simulink model "Assignment1"  (R2020a)
settings: Solver=FixedStepAuto  StartTime=0.0  StopTime=10.0  FixedStep=1e-3  RelTol=1e-3  EnableMultiTasking=on
undefined symbols (not defined in the file or in its folder): D0, D1, D10, D11, D12, D13, D2, D3, D4, D5, D6, D7, D8, D9, PTA0, PTA1, PTA2, PTB23, PTB9, PTC16, PTC17, PTC2, PTC3, PTC4, PTD0, PTD1, PTD2, PTD3
libraries: frdmk64flib x24
settings Model: ExtModeTrigDuration=5  Creator=iceca  LastModifiedBy=iceca
settings OptimizationCC: EnhancedBackFolding=on  PassReuseOutputArgsAs=Individual arguments  ZeroExternalMemoryAtStartup=off  ZeroInternalMemoryAtStartup=off  MaxStackSize=64  OptimizeBlockOrder=speed  DifferentSizesBufferReuse=on  OptimizationCustomize=off  EfficientTunableParamExpr=on
settings DebuggingCC: ParameterTunabilityLossMsg=error
settings HardwareCC: ProdBitPerPointer=32  ProdBitPerSizeT=32  ProdBitPerPtrDiffT=32  ProdLargestAtomicInteger=Long  ProdLargestAtomicFloat=Double  ProdWordSize=32  ProdHWDeviceType=ARM Compatible->ARM Cortex
settings SFSimCC: MATLABDynamicMemAlloc=off
settings RTWCC: SystemTargetFile=ert.tlc  HardwareBoard=NXP FRDM-K64F  TemplateMakefile=ert_default_tmf  Toolchain=GNU Tools for ARM Embedded Processors
settings CodeAppCC: ForceParamTrailComments=on  IgnoreCustomStorageClasses=off  OperatorAnnotations=on  SimulinkDataObjDesc=on  SFDataObjDesc=on  InsertBlockDesc=on

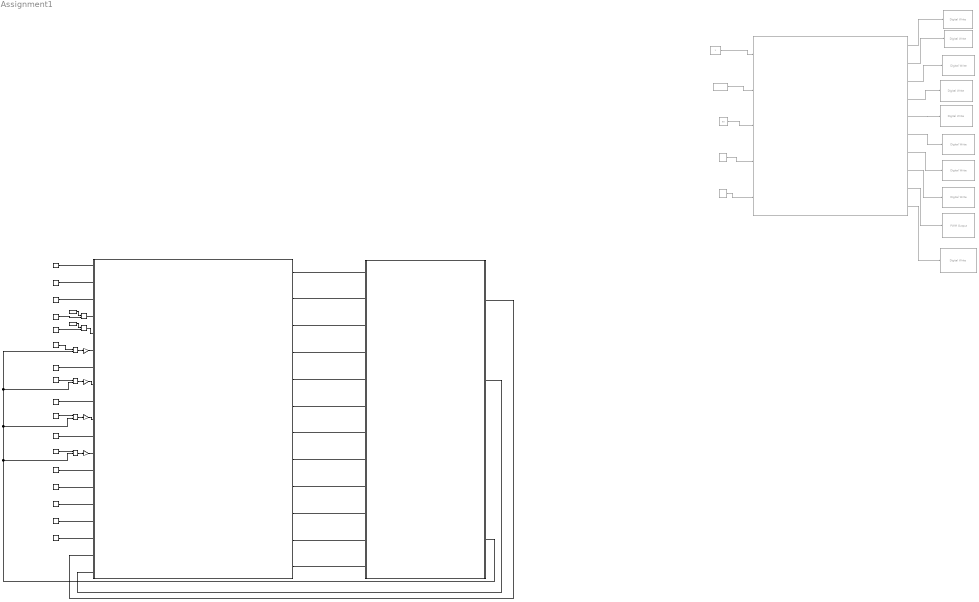
== system Assignment1 ==
  note: Domain: OFF, or percentage
      | in the set (3, 6, 9, 12, 15, 18, 21,25)
  note: Units: pace per minute(ppm)
  note: Domain: 1=Atrial, 2=Ventricular
  note: HARDWARE
  note: Domain: 0=None, 1=Atrial, 2=Ventricular
  note: Domain: 0=None, 2=Inhibited
  note: Units: V
  note: Units: msec
  note: Units: V
  note: Units: msec
  note: Units: V
  note: Units: msec
  note: Units: msec
  note: Units: V
  note: Units: msec
  note: Domain:true, false
  note: Units: msec
  note: Units: pace per minute(ppm)
  note: STATEFLOW
  ARP : Constant  Value=250
  Atrial_Amplitude : Constant  Value=1.5
  Atrial_Pulse_Width : Constant  Value=20
  Atrial_Sensitivity : Constant  Value=3.5
  Chart : Stateflow chart  Commented=on  TreatAsAtomicUnit=on
  Chart1 : Stateflow chart  TreatAsAtomicUnit=on
  Constant24 : Constant  Commented=on  Value=60
  Constant25 : Constant  Commented=on  Value=3.7
  Constant26 : Constant  Commented=on  Value=120
  Constant27 : Constant  Commented=on  Value=10
  Constant28 : Constant  Commented=on
  Digital Write24 : frdmk64flib/Digital Write  Commented=on  Whichpin=PTB9 (D2)
  Digital Write25 : frdmk64flib/Digital Write  Commented=on  Whichpin=PTD0 (D10)
  Digital Write26 : frdmk64flib/Digital Write  Commented=on  Whichpin=PTA0 (D8)
  Digital Write27 : frdmk64flib/Digital Write  Commented=on  Whichpin=PTD2 (D11)
  Digital Write28 : frdmk64flib/Digital Write  Commented=on  Whichpin=PTB23 (D4)
  Digital Write29 : frdmk64flib/Digital Write  Commented=on  Whichpin=PTC3 (D7)
  Digital Write30 : frdmk64flib/Digital Write  Commented=on  Whichpin=PTC4 (D9)
  Digital Write31 : frdmk64flib/Digital Write  Commented=on  Whichpin=PTD3 (D12)
  Digital Write32 : frdmk64flib/Digital Write  Commented=on  Whichpin=BLUE_LED
  Divide{,1..5} (6 alike) : Product  Inputs=*/
  Gain{,1..3} (4 alike) : Gain  Gain=100
  Hysterisis : Constant  Value=0
  Hysterisis Escape Interval : Constant  Value=10
  Lower_Rate_Limit : Constant  Value=60
  Mode_Chamber_Paced : Constant  Value=2
  Mode_Chamber_Sensed : Constant  Value=2
  Mode_Response : Constant  Value=2
  PVARP : Constant  Value=250
  PWM Output : frdmk64flib/PWM Output  Commented=on  Whichpin=PTA2 (D5)  InitialFrequency=2000  InitialDutyCycle=50
  Rate_Smoothing : Constant
  Subsystem : Subsystem
  Upper_Rate_Limit : Constant  Value=120
  VRP : Constant  Value=250
  Ventricular_Amplitude : Constant  Value=4
  Ventricular_Pulse_Width : Constant  Value=10
  Ventricular_Sensitivity : Constant  Value=4
  msec/minute : Constant  Value=60000
  msec/minute 1 : Constant  Value=60000
  wires:
  Chart/1(PACE_CHARGE_CTRL_D2) -> Digital Write24/1
  Chart/2(PACE_GND_CTRL_D10) -> Digital Write25/1
  Chart/3(ATR_PACE_CTRL_D8) -> Digital Write26/1
  Chart/4(ATR_GND_CTRL_D11) -> Digital Write27/1
  Chart/5(Z_ATR_CTRL_D4) -> Digital Write28/1
  Chart/6(Z_VENT_CTRL_D7) -> Digital Write29/1
  Chart/7(VENT_GND_CTRL_D12) -> Digital Write31/1
  Chart/8(VENT_PACE_CTRL_D9) -> Digital Write30/1
  Chart/9(PACING_REF_PWM_D5) -> PWM Output/1
  Constant28/1 -> Chart/1(Pacing_Mode)
  Constant25/1 -> Chart/5(Pulse_Amplitude)
  Constant26/1 -> Chart/4(Upper_Rate_Limit)
  Constant24/1 -> Chart/3(Lower_Rate_Limit)
  Constant27/1 -> Chart/2(Pulse_Width)
  Chart/10(LED_RED) -> Digital Write32/1
  Gain1/1 -> Chart1/10(Atrial_Amplitude)
  VRP/1 -> Chart1/9(VRP)
  Atrial_Sensitivity/1 -> Divide3/1
  Divide2/1 -> Gain1/1
  Divide1/1 -> Gain2/1
  Atrial_Amplitude/1 -> Divide2/1
  Ventricular_Amplitude/1 -> Divide/1
  Ventricular_Sensitivity/1 -> Divide1/1
  Mode_Chamber_Paced/1 -> Chart1/1(Mode_Chamber_Paced)
  Divide3/1 -> Gain3/1
  Gain3/1 -> Chart1/12(Atrial_Sensitivity)
  Gain2/1 -> Chart1/8(Ventricular_Sensitivity)
  Mode_Response/1 -> Chart1/3(Mode_Response)
  Subsystem/4(VOLTAGE_LOGIC_LEVEL) -> Divide3/2, Divide2/2, Divide1/2, Divide/2
  Ventricular_Pulse_Width/1 -> Chart1/7(Ventricular_Pulse_Width)
  Rate_Smoothing/1 -> Chart1/15(Rate_Smoothing)
  Divide/1 -> Gain/1
  Mode_Chamber_Sensed/1 -> Chart1/2(Mode_Chamber_Sensed)
  Atrial_Pulse_Width/1 -> Chart1/11(Atrial_Pulse_Width)
  Hysterisis/1 -> Chart1/16(Hysterisis)
  ARP/1 -> Chart1/13(ARP)
  Gain/1 -> Chart1/6(Ventricular_Amplitude)
  PVARP/1 -> Chart1/14(PVARP)
  msec/minute/1 -> Divide4/1
  Lower_Rate_Limit/1 -> Divide4/2
  Divide4/1 -> Chart1/4(Lower_Rate_Limit)
  Upper_Rate_Limit/1 -> Divide5/2
  msec/minute 1/1 -> Divide5/1
  Divide5/1 -> Chart1/5(Upper_Rate_Limit)
  Hysterisis Escape Interval/1 -> Chart1/17(Hysterisis_Escape_Interval)
  Chart1/1(PACE_CHARGE_CTRL) -> Subsystem/1(PACE_CHARGE_CTRL)
  Chart1/2(PACE_GND_CTRL) -> Subsystem/2(PACE_GND_CTRL)
  Chart1/3(PACING_REF_PWM) -> Subsystem/3(PACING_REF_PWM)
  Chart1/4(VENT_PACE_CTRL) -> Subsystem/4(VENT_PACE_CTRL)
  Chart1/5(ATR_PACE_CTRL) -> Subsystem/5(ATR_PACE_CTRL)
  Chart1/6(ATR_GND_CTRL) -> Subsystem/6(ATR_GND_CTRL)
  Chart1/7(Z_ATR_CTRL) -> Subsystem/7(Z_ATR_CTRL)
  Chart1/8(Z_VENT_CTRL) -> Subsystem/8(Z_VENT_CTRL)
  Chart1/9(VENT_GND_CTRL) -> Subsystem/9(VENT_GND_CTRL)
  Chart1/10(FRONT_END_CTRL) -> Subsystem/10(FRONT_END_CTRL)
  Chart1/11(ATR_CMP_REF_PWM) -> Subsystem/11(ATR_CMP_REF_PWM)
  Chart1/12(VENT_CMP_REF_PWM) -> Subsystem/12(VENT_CMP_REF_PWM)
  Subsystem/1(VENT_CMP_DETECT) -> Chart1/18(ATR_CMP_DETECT)
  Subsystem/2(ATR_CMP_DETECT) -> Chart1/19(VENT_CMP_DETECT)

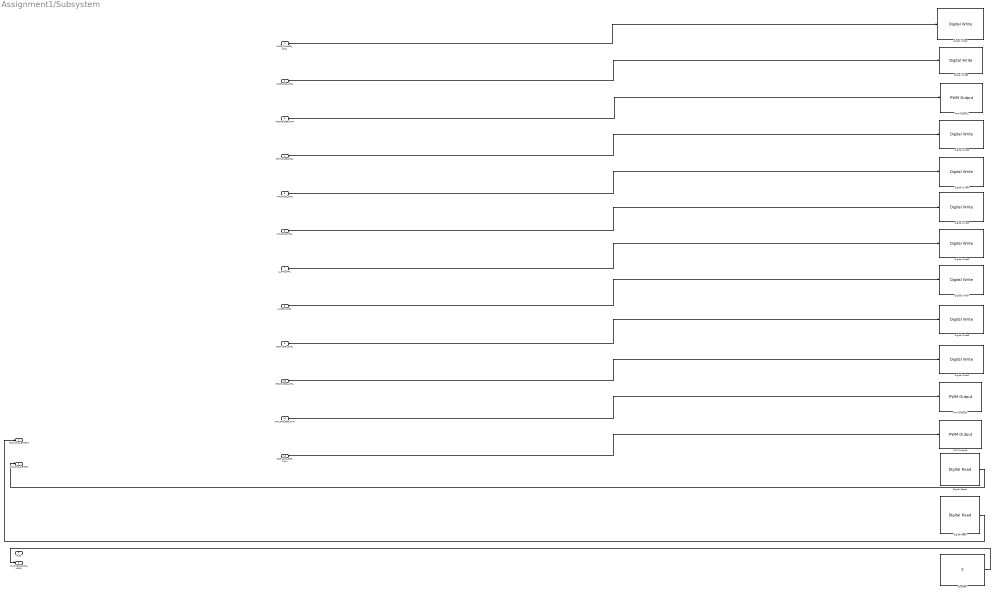
== system Assignment1/Subsystem ==
  PACE_CHARGE_CTRL : Inport
  PACE_GND_CTRL : Inport  Port=2
  PACING_REF_PWM : Inport  Port=3
  VENT_PACE_CTRL : Inport  Port=4
  ATR_PACE_CTRL : Inport  Port=5
  ATR_GND_CTRL : Inport  Port=6
  Z_ATR_CTRL : Inport  Port=7
  Z_VENT_CTRL : Inport  Port=8
  VENT_GND_CTRL : Inport  Port=9
  FRONT_END_CTRL : Inport  Port=10
  ATR_CMP_REF_PWM : Inport  Port=11
  VENT_CMP_REF_PWM : Inport  Port=12
  Constant : Constant  Value=5
  Digital Read : frdmk64flib/Digital Read  Whichpin=PTC16 (D0)  SampleTime=-1
  Digital Read1 : frdmk64flib/Digital Read  Whichpin=PTC17 (D1)  SampleTime=-1
  Digital Write1 : frdmk64flib/Digital Write  Whichpin=PTD1 (D13)
  Digital Write2 : frdmk64flib/Digital Write  Whichpin=PTB9 (D2)
  Digital Write3 : frdmk64flib/Digital Write  Whichpin=PTD0 (D10)
  Digital Write4 : frdmk64flib/Digital Write  Whichpin=PTA0 (D8)
  Digital Write5 : frdmk64flib/Digital Write  Whichpin=PTD2 (D11)
  Digital Write6 : frdmk64flib/Digital Write  Whichpin=PTB23 (D4)
  Digital Write7 : frdmk64flib/Digital Write  Whichpin=PTC3 (D7)
  Digital Write8 : frdmk64flib/Digital Write  Whichpin=PTC4 (D9)
  Digital Write9 : frdmk64flib/Digital Write  Whichpin=PTD3 (D12)
  PWM Output1 : frdmk64flib/PWM Output  Whichpin=PTA2 (D5)  InitialFrequency=2000  InitialDutyCycle=0
  PWM Output2 : frdmk64flib/PWM Output  Whichpin=PTC2 (D6)  InitialFrequency=2000  InitialDutyCycle=0
  PWM Output3 : frdmk64flib/PWM Output  Whichpin=PTA1 (D3)  InitialFrequency=2000  InitialDutyCycle=0
  VENT_CMP_DETECT : Outport
  ATR_CMP_DETECT : Outport  Port=2
  Out3 : Outport  Port=3
  VOLTAGE_LOGIC_LEVEL : Outport  Port=4
  wires:
  PACING_REF_PWM/1 -> PWM Output1/1
  VENT_GND_CTRL/1 -> Digital Write9/1
  PACE_GND_CTRL/1 -> Digital Write3/1
  ATR_GND_CTRL/1 -> Digital Write5/1
  ATR_CMP_REF_PWM/1 -> PWM Output2/1
  VENT_PACE_CTRL/1 -> Digital Write8/1
  Digital Read1/1 -> ATR_CMP_DETECT/1
  Digital Read/1 -> VENT_CMP_DETECT/1
  VENT_CMP_REF_PWM/1 -> PWM Output3/1
  Z_VENT_CTRL/1 -> Digital Write7/1
  Z_ATR_CTRL/1 -> Digital Write6/1
  PACE_CHARGE_CTRL/1 -> Digital Write2/1
  ATR_PACE_CTRL/1 -> Digital Write4/1
  FRONT_END_CTRL/1 -> Digital Write1/1
  Constant/1 -> VOLTAGE_LOGIC_LEVEL/1

== stateflow chart Assignment1/Chart1 ==
  note: |
  note: |
  note: 3 Sections: Atrial only States | Common States | Ventricular only States
  note: |
  note: |
  state Charging_C22
    entry:
    ATR_PACE_CTRL   = LOW;
    VENT_PACE_CTRL = LOW;
  note: Phase 1:
      | Charging Capacitors
  state Atrial_Charge
    entry:
    PACING_REF_PWM = Atrial_Amplitude;
  state Ventricular_Charge
    entry:
    PACING_REF_PWM = Ventricular_Amplitude;
  note: ----------------------------------------------------------------------------------
  state Discharging_C21_and_Pace_Interval_Calculations
    entry:
    PACE_CHARGE_CTRL = HIGH;
    %Discharging C21
    PACE_GND_CTRL=HIGH;
    VENT_PACE_CTRL=LOW;
    Z_ATR_CTRL= LOW;
    Z_VENT_CTRL = LOW;
    ATR_PACE_CTRL = LOW;
    Pace_Interval = Lower_Rate_Limit;
    if Hysterisis == HIGH
    Pace_Interval = Pace_Interval + Hysterisis_Escape_Interval;
    end
  note: Phase 2:
      | Discharging Capacitors
  state Atrial_Discharge
    entry:
    ATR_GND_CTRL= HIGH;
    VENT_GND_CTRL= LOW;
    Pace_Interval =Pace_Interval-Atrial_Pulse_Width;
  state Ventricular_Discharge
    entry:
    ATR_GND_CTRL = LOW;
    VENT_GND_CTRL = HIGH;
    Pace_Interval =Pace_Interval -Ventricular_Pulse_Width;
  note: ---------------------------------------------------------------------------------
  state Atrial_Sensing
    entry:
    FRONT_END_CTRL = HIGH;
    ATR_CMP_REF_PWM= Atrial_Sensitivity;
  state Ventricular_Sensing
    entry:
    FRONT_END_CTRL = HIGH;
    VENT_CMP_REF_PWM = Ventricular_Sensitivity;
  note: Phase 3:
      | Sensing
  state No_Natural_Activity_Sensed
  note: ----------------------------------------------------------------------------------
  state Pacing_Begin
    entry:
    PACE_CHARGE_CTRL = LOW;
    PACE_GND_CTRL = HIGH;
  note: Phase 4:
      | Pacing
  state Ventricular_Pacing
    entry:
    ATR_PACE_CTRL = LOW;
  state Atrial_Pacing
    entry:
    VENT_PACE_CTRL = LOW;
  state Pacing
    entry:
    ATR_GND_CTRL =LOW;
    Z_ATR_CTRL = LOW;
    Z_VENT_CTRL = LOW;
    VENT_GND_CTRL = LOW;
  state Vent_Pacing_2
    entry:
    VENT_PACE_CTRL =HIGH;
  state Atrial_Pacing_2
    entry:
    ATR_PACE_CTRL =HIGH;
  Vent_Pacing_2 -> Charging_C22 : [after(Ventricular_Pulse_Width,msec)]
  Atrial_Pacing_2 -> Charging_C22 : [after(Atrial_Pulse_Width,msec)]
  Ventricular_Sensing -> Charging_C22 [order 2] : [Mode_Response==2 &&  VENT_CMP_DETECT==true && after(VRP, msec)]
  Atrial_Sensing -> Charging_C22 [order 2] : [Mode_Response==2 && after(ARP, msec) && ATR_CMP_DETECT==HIGH]
  (default) -> Charging_C22
  Charging_C22 -> Atrial_Charge [order 2] : [Mode_Chamber_Paced==1]
  Charging_C22 -> Ventricular_Charge [order 1] : [Mode_Chamber_Paced==2]
  Atrial_Charge -> Discharging_C21_and_Pace_Interval_Calculations
  Ventricular_Charge -> Discharging_C21_and_Pace_Interval_Calculations
  Discharging_C21_and_Pace_Interval_Calculations -> Ventricular_Discharge [order 2] : [Mode_Chamber_Paced==2]
  Discharging_C21_and_Pace_Interval_Calculations -> Atrial_Discharge [order 1] : [Mode_Chamber_Paced==1]
  Atrial_Discharge -> Atrial_Sensing [order 2] : [Mode_Chamber_Sensed==1]
  Atrial_Discharge -> No_Natural_Activity_Sensed [order 1] : [Mode_Chamber_Sensed==0 && after(Pace_Interval, msec)]
  Ventricular_Discharge -> No_Natural_Activity_Sensed [order 2] : [Mode_Chamber_Sensed==0 && after(Pace_Interval, msec)]
  Ventricular_Discharge -> Ventricular_Sensing [order 1] : [Mode_Chamber_Sensed==2]
  Atrial_Sensing -> No_Natural_Activity_Sensed [order 1] : [after(Pace_Interval,msec)]
  Ventricular_Sensing -> No_Natural_Activity_Sensed [order 1] : [after(Pace_Interval,msec)]
  No_Natural_Activity_Sensed -> Pacing_Begin
  Pacing_Begin -> Ventricular_Pacing [order 1] : [Mode_Chamber_Paced==2]
  Pacing_Begin -> Atrial_Pacing [order 2] : [Mode_Chamber_Paced==1]
  Atrial_Pacing -> Pacing
  Ventricular_Pacing -> Pacing
  Pacing -> Atrial_Pacing_2 [order 2] : [Mode_Chamber_Paced==1]
  Pacing -> Vent_Pacing_2 [order 1] : [Mode_Chamber_Paced==2]
  data: Mode_Chamber_Paced input; Mode_Chamber_Sensed input; Mode_Response input; PACE_CHARGE_CTRL output; PACE_GND_CTRL output; PACING_REF_PWM output; VENT_PACE_CTRL output; ATR_PACE_CTRL output; ATR_GND_CTRL output; Z_ATR_CTRL output; Z_VENT_CTRL output; VENT_GND_CTRL output; Lower_Rate_Limit input; Upper_Rate_Limit input; HIGH local boolean =true; LOW local boolean =false; Ventricular_Amplitude input; Ventricular_Pulse_Width input; Ventricular_Sensitivity input; VRP input; Atrial_Amplitude input; Atrial_Pulse_Width input; Atrial_Sensitivity input; ARP input; PVARP input; Rate_Smoothing input; FRONT_END_CTRL output; ATR_CMP_REF_PWM output; VENT_CMP_REF_PWM output; Hysterisis input; Hysterisis_Escape_Interval input; ATR_CMP_DETECT input; VENT_CMP_DETECT input; Pace_Interval local

== stateflow chart Assignment1/Chart ==
  state AV_Pacing_state_2
    entry:
    LED_RED = LOW;
    %PACING_REF_PWM_D5 = 75;
    %PACE_CHARGE_CTRL_D2 = LOW;
    %VENT_PACE_CTRL_D9 = HIGH;
    %VENT_GND_CTRL_D12 = LOW;
    %PACE_GND_CTRL_D10 = HIGH;
    %Z_VENT_CTRL_D7 = LOW;
    PACE_CHARGE_CTRL_D2 = LOW;
    PACE_GND_CTRL_D10 = HIGH;
    ATR_PACE_CTRL_D8 = LOW;
    ATR_GND_CTRL_D11 =LOW;
    Z_ATR_CTRL_D4 = LOW;
    Z_VENT_CTRL_D7 = LOW;
    VENT_GND_CTRL_D12 = LOW;
    if Pacing_Mode == 1
    VENT_PACE_CTRL_D9 =HIGH;
    else
    VENT_PACE_CTRL_D9 =LOW;
    ATR_PACE_CTRL_D8 =HIGH;
    end
  state Discharching_C21_and_Charging_C22
    entry:
    %charging C22
    LED_RED=HIGH;
    ATR_PACE_CTRL_D8   = LOW;
    VENT_PACE_CTRL_D9 = LOW;
    PACING_REF_PWM_D5 = Pulse_Amplitude*20;
    PACE_CHARGE_CTRL_D2 = HIGH;
    %discharching C21
    PACE_GND_CTRL_D10=HIGH;
    VENT_PACE_CTRL_D9=LOW;
    Z_ATR_CTRL_D4 = LOW;
    Z_VENT_CTRL_D7 = LOW;
    ATR_PACE_CTRL_D8 = LOW;
    if Pacing_Mode == 1
    VENT_GND_CTRL_D12 = HIGH;
    else
    ATR_GND_CTRL_D11 = HIGH;
    VENT_GND_CTRL_D12= LOW;
    end
    Rate = 60000/40 - Pulse_Width;
  (default) -> Discharching_C21_and_Charging_C22
  Discharching_C21_and_Charging_C22 -> AV_Pacing_state_2 : [after(300, msec)]
  AV_Pacing_state_2 -> Discharching_C21_and_Charging_C22 : [after(Pulse_Width, msec)]
  data: PACE_CHARGE_CTRL_D2 output; PACE_GND_CTRL_D10 output; ATR_PACE_CTRL_D8 output; ATR_GND_CTRL_D11 output; Z_ATR_CTRL_D4 output; Z_VENT_CTRL_D7 output; VENT_GND_CTRL_D12 output; VENT_PACE_CTRL_D9 output; Pacing_Mode input; PACING_REF_PWM_D5 output; Pulse_Width input double; avgRate local double; Lower_Rate_Limit input double; Upper_Rate_Limit input; Rate local double; Pulse_Amplitude input; HIGH local boolean =true; LOW local boolean =false; LED_RED output
